simulink model "dc_motor_control"  (R2015a)
settings: Solver=ode45  StartTime=0.0  StopTime=10.0  RelTol=1e-3
settings Model: Creator=Suwandi Dwi S  LastModifiedBy=Suwandi Dwi S

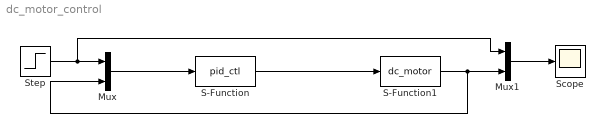
== system dc_motor_control ==
  Mux : Mux  Inputs=2
  Mux1 : Mux  Inputs=2
  S-Function : S-Function  FunctionName=pid_ctl
  S-Function1 : S-Function  FunctionName=dc_motor
  Scope : Scope
  Step : Step  After=10  SampleTime=0
  wires:
  Mux1/1 -> Scope/1
  S-Function1/1 -> Mux/2, Mux1/2
  S-Function/1 -> S-Function1/1
  Mux/1 -> S-Function/1
  Step/1 -> Mux1/1, Mux/1
